simulink model "bang_bang_sim"  (R2020b)
settings: Solver=VariableStepAuto  StartTime=0.0  StopTime=60  MaxStep=1e-3  RelTol=1e-3
libraries: simulink x1
settings Model: Creator=remy  LastModifiedBy=remy
settings SolverCC: ZeroCrossAlgorithm=Adaptive
settings DebuggingCC: IgnoredZcDiagnostic=none

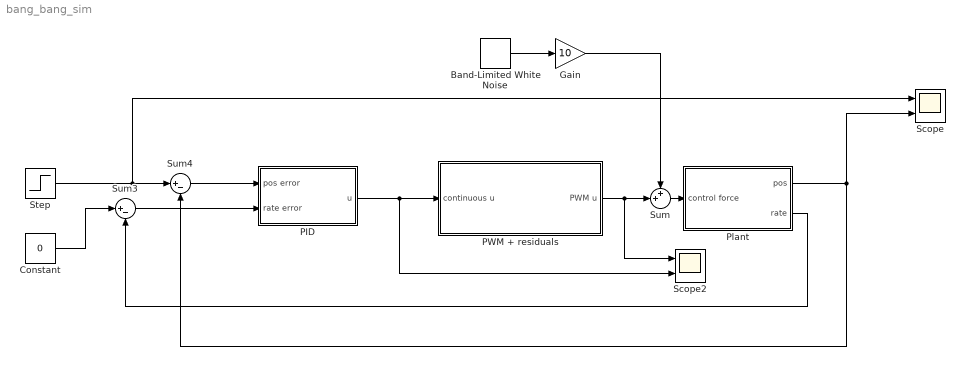
== system bang_bang_sim ==
  Band-Limited White Noise : simulink/Sources/Band-Limited White Noise  Cov=[0.1]  Ts=1e-3  seed=[23341]
  Constant : Constant  Value=0
  Gain : Gain  Gain=10
  PID : Subsystem
  PWM + residuals : Subsystem
  Plant : Subsystem
  Scope : Scope  NumInputPorts=2
  Scope2 : Scope  NumInputPorts=2
  Step : Step  Time=20  After=10  SampleTime=0
  Sum : Sum  Inputs=++|
  Sum3 : Sum  Inputs=|+-
  Sum4 : Sum  Inputs=|+-
  wires:
  Step/1 -> Scope/1, Sum4/1
  Constant/1 -> Sum3/1
  Sum4/1 -> PID/1(pos error)
  Sum3/1 -> PID/2(rate error)
  PWM + residuals/1(PWM u) -> Sum/2, Scope2/1
  PID/1(u) -> PWM + residuals/1(continuous u), Scope2/2
  Plant/2(rate) -> Sum3/2
  Plant/1(pos) -> Scope/2, Sum4/2
  Band-Limited White Noise/1 -> Gain/1
  Sum/1 -> Plant/1(control force)
  Gain/1 -> Sum/1

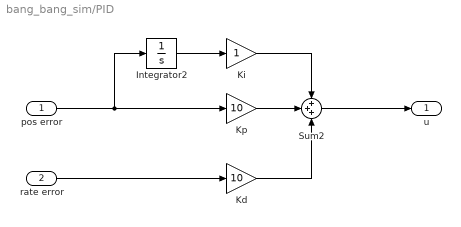
== system bang_bang_sim/PID ==
  pos error : Inport
  rate error : Inport  Port=2
  Integrator2 : Integrator
  Kd : Gain  Gain=10
  Ki : Gain
  Kp : Gain  Gain=10
  Sum2 : Sum  Inputs=+++
  u : Outport
  wires:
  Sum2/1 -> u/1
  rate error/1 -> Kd/1
  Ki/1 -> Sum2/1
  pos error/1 -> Integrator2/1, Kp/1
  Integrator2/1 -> Ki/1
  Kd/1 -> Sum2/3
  Kp/1 -> Sum2/2

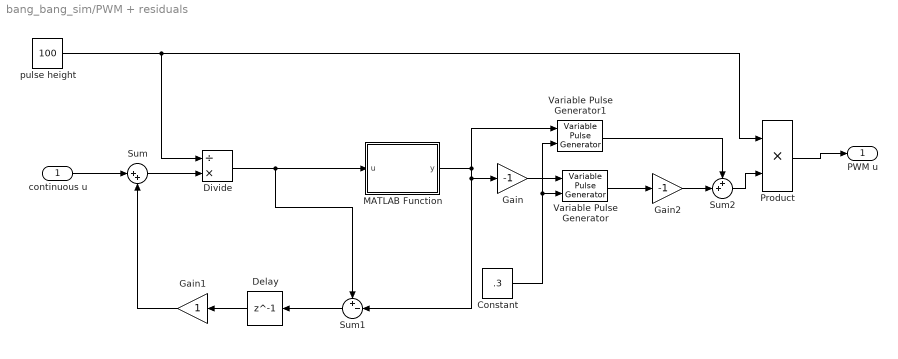
== system bang_bang_sim/PWM + residuals ==
  continuous u : Inport
  Constant : Constant  Value=.3
  Delay : Delay  DelayLength=1
  Divide : Product  Inputs=/*
  Gain : Gain  Gain=-1
  Gain1 : Gain
  Gain2 : Gain  Gain=-1
  MATLAB Function : MATLAB Function  TreatAsAtomicUnit=on
  Product : Product
  Sum : Sum  Inputs=|++
  Sum1 : Sum  Inputs=+-|
  Sum2 : Sum  Inputs=++|
  Variable Pulse Generator : VariablePulseGenerator  AllowZeroPulseWidth=on  SampleTime=0.1
  Variable Pulse Generator1 : VariablePulseGenerator  AllowZeroPulseWidth=on  SampleTime=0.1
  pulse height : Constant  Value=100
  PWM u : Outport
  wires:
  continuous u/1 -> Sum/1
  Delay/1 -> Gain1/1
  Gain1/1 -> Sum/2
  Sum/1 -> Divide/2
  Variable Pulse Generator1/1 -> Sum2/1
  Divide/1 -> Sum1/1, MATLAB Function/1(u)
  Product/1 -> PWM u/1
  MATLAB Function/1(y) -> Variable Pulse Generator1/1, Gain/1, Sum1/2
  pulse height/1 -> Divide/1, Product/1
  Sum1/1 -> Delay/1
  Gain/1 -> Variable Pulse Generator/1
  Variable Pulse Generator/1 -> Gain2/1
  Gain2/1 -> Sum2/2
  Sum2/1 -> Product/2
  Constant/1 -> Variable Pulse Generator/2, Variable Pulse Generator1/2

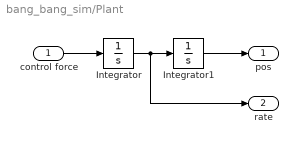
== system bang_bang_sim/Plant ==
  control force : Inport
  Integrator : Integrator
  Integrator1 : Integrator
  pos : Outport
  rate : Outport  Port=2
  wires:
  control force/1 -> Integrator/1
  Integrator1/1 -> pos/1
  Integrator/1 -> rate/1, Integrator1/1

== matlab function bang_bang_sim/PWM + residuals/MATLAB Function ==
  data: u input; y output
function y = fcn(u)

    d1 = .1;
    d2 = .5;
    
    if u < -d2
        y = -d2;
    elseif u < -d1
        y = u;
    elseif u < d1
        y = 0;
    elseif u < d2
        y = u;
    else
        y = d2;
    end

end
